simulink model "motor_io_velocity"  (R2014b)
settings: Solver=ode1  StartTime=0.0  StopTime=inf  FixedStep=Ts  RelTol=1e-3
PostLoadFcn:
  | , if any(exist('dsrtsu_mdlpostloadfcn', 'file') == [2, 3, 6]), try dsrtsu_mdlpostloadfcn('Execute', bdroot); catch fprintf('Error in PostLoadFcn (dsrtsu_mdlpostloadfcn) for model "%s":\n %s\n', bdroot, lasterr); end, end,
values from neighbouring files (symbols this model uses):
  F_c = 1.5e-3    (= 0.0015)    [continuous_design.m]    (also in workshop1.m)
  Gfb_d = c2d(S/R, Ts, 'tustin')    [continuous_design.m]    (also in workshop1.m = minreal(c2d(S/R, Ts, 'tustin')))
  Gff_d = c2d(T/R, Ts, 'tustin')    [continuous_design.m]    (also in workshop1.m = minreal(c2d(T/R, Ts, 'tustin')))
  J1 = 0.0006    [continuous_design.m]    (also in workshop1.m)
  motor = motor_pars    [continuous_design.m]    (also in workshop1.m)
  n = 5    [continuous_design.m]    (also in workshop1.m)
  R_vector = [1 0]    [workshop1.m]
  S_vector = [s1 s2]    [workshop1.m]
  T_vector = t0*[1 omega2]    [workshop1.m]
  Ts = 2*pi/ws    (= 0.0199466200228)    [continuous_design.m]    (also in pbutest.m = 0.0108705628152; workshop1.m = Ts_p)
libraries: rtilib1104 x5, simulink x1
settings Model: DSRTSU_INTERNAL_RTI_VER=450  DSRTSU_INTERNAL_RTI_TYPE=rti1104  DSRTSU_INTERNAL_RTIFPGA=40  ExtModeArmWhenConnect=off  BufferReuse=off  Creator=user  LastModifiedBy=es2lab2
settings DataIOCC: SignalLoggingSaveFormat=ModelDataLogs  SaveOutput=off  SignalLoggingName=sigsOut
settings OptimizationCC: BlockReduction=off  ConditionallyExecuteInputs=off  OptimizeBlockIOStorage=off  BufferReuse=off  GlobalBufferReuse=off  ExpressionFolding=off  ExpressionDepthLimit=2147483647  LocalBlockOutputs=off  InitFltsAndDblsToZero=on
settings DebuggingCC: SaveWithParameterizedLinksMsg=none  UnderspecifiedInitializationDetection=Classic  MergeDetectMultiDrivingBlocksExec=none  SignalResolutionControl=TryResolveAllWithWarning  SolverPrmCheckMsg=none  MultiTaskDSMMsg=warning  MultiTaskCondExecSysMsg=none  FcnCallInpInsideContextMsg=UseLocalSettings  UnconnectedInputMsg=none  UnconnectedOutputMsg=none  StateNameClashWarn=warning
settings HardwareCC: ProdIntDivRoundTo=Zero  ProdEndianess=BigEndian  ProdHWDeviceType=Generic->Custom  TargetIntDivRoundTo=Zero  TargetEndianess=BigEndian  TargetHWDeviceType=Generic->Custom
settings RTWCC: SystemTargetFile=rti1104.tlc  MakeCommand=make_rti  TemplateMakefile=rti1104.tmf  Description=dSPACE DS1104 Hardware Platform  RetainRTWFile=on  ProcessScript=rti1104_make_rtw_hook  IncludeERTFirstTime=on
settings STFCustomTargetCC: TargetFcnLib=ansi_tfl_tmw.mat  ParMdlRefBuildCompliant=on  GeneratePreprocessorConditionals=Disable all  SystemTargetFile=rti1104.tlc
settings GRTTargetCC: TargetFcnLib=ansi_tfl_tmw.mat  CompOptLevelCompliant=off  ConcurrentExecutionCompliant=off  CombineOutputUpdateFcns=off  MatFileLogging=off  CPPClassGenCompliant=off  GRTInterface=on  ExtModeMexFile=noextcomm

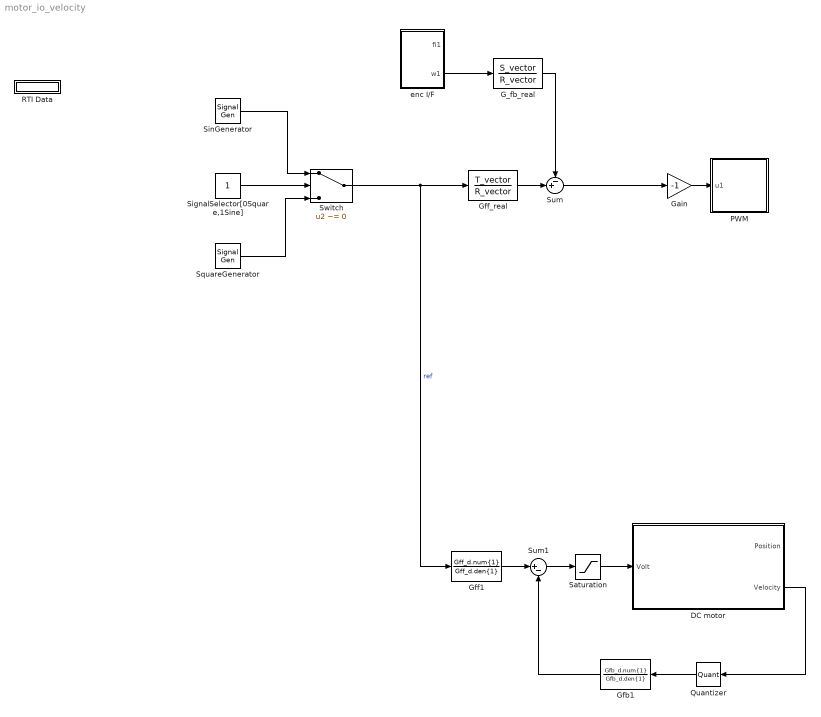
== system motor_io_velocity ==
  DC motor : Subsystem
  G_fb_real : DiscreteTransferFcn  Numerator=S_vector  Denominator=R_vector  SampleTime=Ts
  Gain : Gain  Gain=-1
  Gfb1 : DiscreteTransferFcn  Numerator=Gfb_d.num{1}  Denominator=Gfb_d.den{1}  SampleTime=Ts
  Gff1 : DiscreteTransferFcn  Numerator=Gff_d.num{1}  Denominator=Gff_d.den{1}  SampleTime=Ts
  Gff_real : DiscreteTransferFcn  Numerator=T_vector  Denominator=R_vector  SampleTime=Ts
  PWM : Subsystem
  Quantizer : Quantizer  QuantizationInterval=quant
  RTI Data : Subsystem  Tag=struct('RTIDataServer',struct('RTIDataServerVs','2','RTIModelDescription','struct(''main'',''motor_io_velocity'',''sub'','''',''isMp'',0)'))  LoadFcn="if exist('rtidc'), try,  rtidc('DataHostBlockClbLoad', gcbh); catch, disp(['Warning: ''LoadFcn'' for RTI Data block failed: ' lasterr]); end, end,"  mask(RTI_DATA_HOST){}
      mask help:
      | RTI Data Block.
      | This block is used by RTI to store internal model-dependent data.
      | Please keep this block on the root level of the model. Deleting this block will result in data loss.
      |
      | NEVER DELETE OR COPY THIS BLOCK!
      settings: CopyFcn="if exist('rtidc'), try,  rtidc('DataHostBlockClbCopy', gcbh); catch, disp(['Warning: ''CopyFcn'' for RTI Data block failed: ' lasterr]); end, end,"  DeleteFcn="if exist('rtidc'), try,  rtidc('DataHostBlockClbDelete', gcbh); catch, disp(['Warning: ''DeleteFcn'' for RTI Data block failed: ' lasterr]); end, end,"  ModelCloseFcn="if exist('rtidc'), try,  rtidc('DataHostBlockClbModelClose', gcbh); catch, disp(['Warning: ''ModelCloseFcn'' for RTI Data block failed: ' lasterr]); end, end,"  PreSaveFcn="if exist('rtidc'), try,  rtidc('DataHostBlockClbPreSave', gcbh); catch, disp(['Warning: ''PreSaveFcn'' for RTI Data block failed: ' lasterr]); end, end,"  PostSaveFcn="if exist('rtidc'), try,  rtidc('DataHostBlockClbPostSave', gcbh); catch, disp(['Warning: ''PostSaveFcn'' for RTI Data block failed: ' lasterr]); end, end,"  NameChangeFcn="if exist('rtidc'), try,  rtidc('DataHostBlockClbNameChange', gcbh); catch, disp(['Warning: ''NameChangeFcn'' for RTI Data block failed: ' lasterr]); end, end,"
      mask Help:
      | RTI Data Block.
      | This block is used by RTI to store internal model-dependent data.
      | Please keep this block on the root level of the model. Deleting this block will result in data loss.
      | 
      | NEVER DELETE OR COPY THIS BLOCK!
      mask Display:
      | text(0.5, 0.5, 'RTI Data', 'HorizontalAlignment', 'center');
      | plot([1 0]);
  Saturation : Saturate  UpperLimit=24  LowerLimit=-24
  SignalSelector[0Square,1Sine] : Constant
  SinGenerator : SignalGenerator  Amplitude=0  Units=rad/sec
  SquareGenerator : SignalGenerator  WaveForm=square  Amplitude=0  Units=rad/sec
  Sum : Sum  Inputs=-+|
  Sum1 : Sum  Inputs=|+-
  Switch : Switch  Criteria=u2 ~= 0
  enc I/F : Subsystem
  wires:
  SinGenerator/1 -> Switch/1
  SquareGenerator/1 -> Switch/3
  SignalSelector[0Square,1Sine]/1 -> Switch/2
  Gain/1 -> PWM/1(u1)
  Switch/1 -> Gff1/1, Gff_real/1  "ref"
  ? -> ?
  Gff_real/1 -> Sum/2
  Gff1/1 -> Sum1/1
  Sum1/1 -> Saturation/1
  Sum/1 -> Gain/1
  Gfb1/1 -> Sum1/2
  DC motor/2(Velocity) -> Quantizer/1
  enc I/F/2(w1) -> G_fb_real/1
  G_fb_real/1 -> Sum/1
  Saturation/1 -> DC motor/1(Volt)
  Quantizer/1 -> Gfb1/1

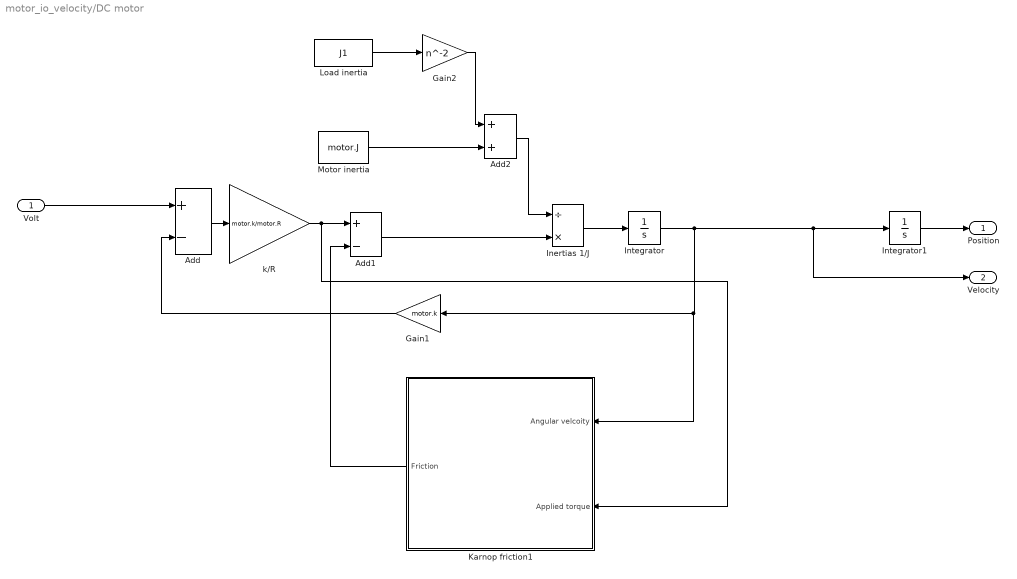
== system motor_io_velocity/DC motor ==
  Volt : Inport
  Add : Sum  Inputs=+-
  Add1 : Sum  Inputs=+-
  Add2 : Sum
  Gain1 : Gain  Gain=motor.k
  Gain2 : Gain  Gain=n^-2
  Inertias 1/J : Product  Inputs=/*
  Integrator : Integrator
  Integrator1 : Integrator
  Karnop friction1 : Subsystem
  Load inertia : Constant  Value=J1
  Motor inertia : Constant  Value=motor.J
  "k/R " : Gain  Gain=motor.k/motor.R
  Position : Outport
  Velocity : Outport  Port=2
  wires:
  Gain1/1 -> Add/2
  Add/1 -> "k/R "/1
  "k/R "/1 -> Karnop friction1/2(Applied torque), Add1/1
  Inertias 1/J/1 -> Integrator/1
  Integrator1/1 -> Position/1
  Add1/1 -> Inertias 1/J/2
  Volt/1 -> Add/1
  Integrator/1 -> Karnop friction1/1(Angular velcoity), Gain1/1, Velocity/1, Integrator1/1
  Motor inertia/1 -> Add2/2
  Load inertia/1 -> Gain2/1
  Gain2/1 -> Add2/1
  Add2/1 -> Inertias 1/J/1
  Karnop friction1/1(Friction) -> Add1/2

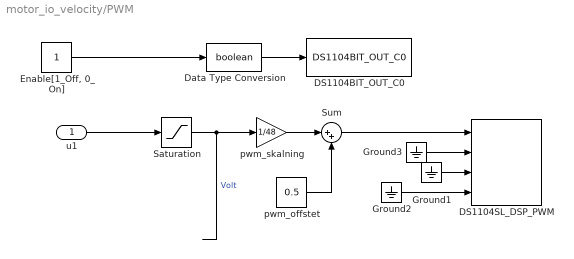
== system motor_io_velocity/PWM ==
  u1 : Inport
  DS1104BIT_OUT_C0 : rtilib1104/DS1104 MASTER PPC/DS1104BIT_OUT_C0  ChannelNo=0  InitValue=1  TermMode=0  TermValue=0  Reserved1=[]  Reserved2=[]  Reserved3=[]  Reserved=[]  DialogFcn=gui1104bit_out  UnitName={'DS1104BIT_OUT_C'}  UnitValues={ 0 }  DSProperties=struct('RTI',struct('Version',uint32(1),'BlockType',struct('isSLSource',uint8(0),'isSLSink',uint8(1),'isHWSource',uint8(0),'isHWSink',uint8(1),'isSetup',uint8(0),'isInline',uint8(1),'isNonInline',uint8(0),'isInterrupt',uint8(0),'isChannelwise',uint8(1)),'IOBoardType','DS1104MASTER','UnitType','BIT','Identifier','BITOUTCH','DialogType','ML','BlockSet','NONE','SlaveProcessor','NONE'))
  DS1104SL_DSP_PWM : rtilib1104/DS1104 SLAVE DSP/DS1104SL_DSP_PWM  Parameters=[]  TDef=[]  BoardType=[]  PwmMode=1  Frequency=20000  InitValue=[0.5 0.5 0.5 0.5]  TermMode=[0 0 0 0]  TermValue=[0.5 0.5 0.5 0.5]  Polarity=[1 1 1 1]  DialogFcn=gui1104sl_dsp_pwm  Reserved1=[]  Reserved2=[]  Reserved3=[]  Reserved4=[]  Revision=[]  UnitName={'DS1104SL_DSP_PWM'}  UnitValues={[]}  DSProperties=struct('RTI',struct('Version',uint32(2),'BlockType',struct('isSLSource',uint8(0),'isSLSink',uint8(1),'isHWSource',uint8(0),'isHWSink',uint8(1),'isSetup',uint8(0),'isInline',uint8(1),'isNonInline',uint8(0),'isInterrupt',uint8(0),'isChannelwise',uint8(0)),'IOBoardType','DS1104SLAVE','UnitType','PWM','Identifier','PWM','DialogType','ML','BlockSet','NONE','SlaveProcessor','F240'))  RTIBlockInterface=struct('InputPortsActive',[1 1 1 1],'InputPortsWidth',int32([1 1 1 1]),'InputPortsName',{{['PWM Channel 1'],['PWM Channel 2'],['PWM Channel 3'],['PWM Channel 4']}},'IWork',{{{'',uint32(4)}}},'DialogFcn','rti1104slavepwmgui','InitLevel',1,'BlockDisplay',{{'','auto'}},'IconTransparency','on','MultiSFcn',4,'BlockName',struct('Token',{{'DS1104SL_DSP_PWM'}}))  RTIBlockParameters=struct('PWMSymmetryMode',{{1,'OFF',[]}},'PWMFrequency',{{'50000','OFF',[]}},'PWMPolarityMode',{{[1 1 1 1 1],'OFF',[]}},'ChannelNo',{{[1 2 3 4],'OFF',[]}},'SuspendModeInit',{{[0 0 0 0 1],'OFF',[]}},'TTLModeInit',{{[2 2 2 2 2],'OFF',[]}},'DutyCycleInitValueCh1',{{'0.5','OFF',[]}},'DutyCycleInitValueCh2',{{'0.5','OFF',[]}},'DutyCycleInitValueCh3',{{'0.5','OFF',[]}},'DutyCycleInitValueCh4',{{'0.5','OFF',[]}},'DutyCycleInitValueCh5',{{'0.5','OFF',[]}},'EnablePWMStop',{{[0 0 0 0 0],'OFF',[]}},'SuspendModeTerm',{{[0 0 0 0 1],'OFF',[]}},'TTLModeTerm',{{[2 2 2 2 2],'OFF',[]}},'DutyCycleTermValueCh1',{{'0.5','OFF',[]}},'DutyCycleTermValueCh2',{{'0.5','OFF',[]}},'DutyCycleTermValueCh3',{{'0.5','OFF',[]}},'DutyCycleTermValueCh4',{{'0.5','OFF',[]}},'DutyCycleTermValueCh5',{{'0.5','OFF',[]}},'TLCFileName',{{'rti1104pwm','OFF',[]}})  RTISFcnParameters=struct('PWMSymmetryMode','double','PWMFrequency','double','PWMPolarityMode','double','ChannelNo','double','SuspendModeInit','double','TTLModeInit','double','DutyCycleInitValueCh1','double','DutyCycleInitValueCh2','double','DutyCycleInitValueCh3','double','DutyCycleInitValueCh4','double','EnablePWMStop','double','SuspendModeTerm','double','TTLModeTerm','double','DutyCycleTermValueCh1','double','DutyCycleTermValueCh2','double','DutyCycleTermValueCh3','double','DutyCycleTermValueCh4','double','TLCFileName','char')  RTIBlockParaDefault=struct('PWMSymmetryMode',1,'PWMFrequency',100,'PWMPolarityMode',[1 1 1 1 1],'ChannelNo',[1 2 3 4],'SuspendModeInit',[1 1 1 1 1],'TTLModeInit',[2 2 2 2 2],'DutyCycleInitValueCh1',0.5,'DutyCycleInitValueCh2',0.5,'DutyCycleInitValueCh3',0.5,'DutyCycleInitValueCh4',0.5,'DutyCycleInitValueCh5',0.5,'EnablePWMStop',[1 1 1 1 0],'SuspendModeTerm',[1 1 1 1 1],'TTLModeTerm',[2 2 2 2 2],'DutyCycleTermValueCh1',0.5,'DutyCycleTermValueCh2',0.5,'DutyCycleTermValueCh3',0.5,'DutyCycleTermValueCh4',0.5,'DutyCycleTermValueCh5',0.5,'TLCFileName','rti1104pwm')
  Data Type Conversion : DataTypeConversion  OutDataTypeStr=boolean  SaturateOnIntegerOverflow=on  RndMeth=Zero
  "Enable[1_Off, 0_On]" : Constant
  Ground1 : Ground
  Ground2 : Ground
  Ground3 : Ground
  Saturation : Saturate  UpperLimit=24  LowerLimit=-24
  Sum : Sum  Inputs=|++  SaturateOnIntegerOverflow=on
  pwm_offstet : Constant  Value=0.5
  pwm_skalning : Gain  Gain=1/48  SaturateOnIntegerOverflow=on  OutDataTypeStr=Inherit: Same as input  ParamDataTypeStr=Inherit: Same as input
  wires:
  "Enable[1_Off, 0_On]"/1 -> Data Type Conversion/1
  Data Type Conversion/1 -> DS1104BIT_OUT_C0/1
  pwm_skalning/1 -> Sum/1
  Sum/1 -> DS1104SL_DSP_PWM/1
  pwm_offstet/1 -> Sum/2
  u1/1 -> Saturation/1
  Ground1/1 -> DS1104SL_DSP_PWM/3
  Ground2/1 -> DS1104SL_DSP_PWM/4
  Ground3/1 -> DS1104SL_DSP_PWM/2
  Saturation/1 -> pwm_skalning/1  "Volt"

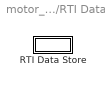
== system motor_io_velocity/RTI Data ==
  RTI Data Store : Subsystem  Tag="struct('public',struct('sub',struct('name',{{'motor_io_velocity'}},'data',{{struct('TH',struct('thTaskInfo',struct('taskType',{'TIMER','HWINT','TMRINT','SWINT','GLINT'},'tasksNumOf',{1,0,0,0,0},'srcIds',{{'TIMERA'},{},{},{},{}},'taskNames',{{['Timer Task 1']},{},{},{},{}})),'th_tc',struct('dataType','TASK','taskGroupId','','taskGroupList',{{}},'taskSchedulingPolicy','FCFS','taskType','TIMER','blkh',-1,'srcId','TIMERA','srcSgnName',['Timer A interrupt'],'srcCpuName','','taskName',['Timer Task 1  [0.0219701] s'],'taskNameDisplayExt','','smplTime',0.021970064966318436,'smplTimeOffs',0,'hasFixedPriority',0,'priority',1,'hasFixedOvc',0,'ovcType',1,'ovcMax',1),'tc_th',struct('dataType','TASK','taskGroupId','','taskGroupList',{{}},'taskSchedulingPolicy','FCFS','taskType','TIMER','blkh',-1,'srcId','TIMERA','srcSgnName',['Timer A interrupt'],'srcCpuName','','taskName',['Timer Task 1  [0.0219701] s'],'taskNameDisplayExt','','smplTime',0.021970064966318436,'smplTimeOffs',0,'hasFixedPriority',0,'priority',1,'hasFixedOvc',0,'ovcType',1,'ovcMax',1))}})),'private',struct('version',struct('dsVer',uint32(2)),'access',struct('modified',['30-Mar-2016 14:28:40'],'type','Model','isPerm',1)))"  mask(RTI_DATA_STORE){}
      mask help:
      | RTI Data Store Block. This block is used by RTI to store internal model dependent data. Deleting this block will result in data loss.
      |
      | NEVER DELETE, COPY, OR MODIFY THIS BLOCK!
      mask Help:
      | RTI Data Store Block. This block is used by RTI to store internal model dependent data. Deleting this block will result in data loss.
      | 
      | NEVER DELETE, COPY, OR MODIFY THIS BLOCK!
      mask Display: text(0.5, 0.5, ' ', 'HorizontalAlignment', 'center');

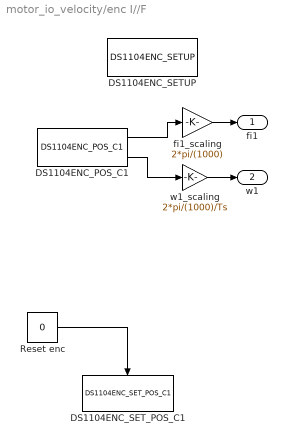
== system motor_io_velocity/enc I//F ==
  DS1104ENC_POS_C1 : rtilib1104/DS1104 MASTER PPC/DS1104ENC_POS_C1  ChannelNo=1  PosValue=0  Reserved1=[]  Reserved2=[]  Reserved3=[]  Reserved4=[]  DialogFcn=gui1104enc_pos  UnitName={'DS1104ENC_POS_C'}  UnitValues={ 1 }  DSProperties=struct('RTI',struct('Version',uint32(1),'BlockType',struct('isSLSource',uint8(1),'isSLSink',uint8(0),'isHWSource',uint8(1),'isHWSink',uint8(0),'isSetup',uint8(0),'isInline',uint8(1),'isNonInline',uint8(0),'isInterrupt',uint8(0),'isChannelwise',uint8(1)),'IOBoardType','DS1104MASTER','UnitType','ENC','Identifier','ENCPOSCH','DialogType','ML','BlockSet','NONE','SlaveProcessor','NONE'))
  DS1104ENC_SETUP : rtilib1104/DS1104 MASTER PPC/DS1104ENC_SETUP  Reserved1=[]  Reserved2=[]  Reserved3=[]  Reserved4=[]  DialogFcn=gui1104enc_setup  UnitName={'DS1104ENC_SETUP'}  UnitValues={ [] }  DSProperties=struct('RTI',struct('Version',uint32(1),'BlockType',struct('isSLSource',uint8(0),'isSLSink',uint8(0),'isHWSource',uint8(0),'isHWSink',uint8(0),'isSetup',uint8(0),'isInline',uint8(1),'isNonInline',uint8(0),'isInterrupt',uint8(0),'isChannelwise',uint8(0)),'IOBoardType','DS1104MASTER','UnitType','ENC','Identifier','ENCSETUP','DialogType','ML','BlockSet','NONE','SlaveProcessor','NONE'))
      settings: SignalType=[1 0]
  DS1104ENC_SET_POS_C1 : rtilib1104/DS1104 MASTER PPC/DS1104ENC_SET_POS_C1  ChannelNo=1  PosValue=0  Reserved1=[]  Reserved2=[]  Reserved3=[]  Reserved4=[]  DialogFcn=gui1104enc_set_pos  UnitName={'DS1104ENC_SET_POS_C'}  UnitValues={ 1 }  DSProperties=struct('RTI',struct('Version',uint32(1),'BlockType',struct('isSLSource',uint8(0),'isSLSink',uint8(1),'isHWSource',uint8(0),'isHWSink',uint8(1),'isSetup',uint8(0),'isInline',uint8(1),'isNonInline',uint8(0),'isInterrupt',uint8(0),'isChannelwise',uint8(1)),'IOBoardType','DS1104MASTER','UnitType','ENC','Identifier','ENCRESET','DialogType','ML','BlockSet','NONE','SlaveProcessor','NONE'))
  Reset enc : Constant  Value=0
  fi1_scaling : Gain  Gain=2*pi/(1000)  SaturateOnIntegerOverflow=on  OutDataTypeStr=Inherit: Same as input  ParamDataTypeStr=Inherit: Same as input
  w1_scaling : Gain  Gain=2*pi/(1000)/Ts  SaturateOnIntegerOverflow=on  OutDataTypeStr=Inherit: Same as input  ParamDataTypeStr=Inherit: Same as input
  fi1 : Outport
  w1 : Outport  Port=2
  wires:
  Reset enc/1 -> DS1104ENC_SET_POS_C1/Trigger
  DS1104ENC_POS_C1/1 -> fi1_scaling/1
  DS1104ENC_POS_C1/2 -> w1_scaling/1
  fi1_scaling/1 -> fi1/1
  w1_scaling/1 -> w1/1

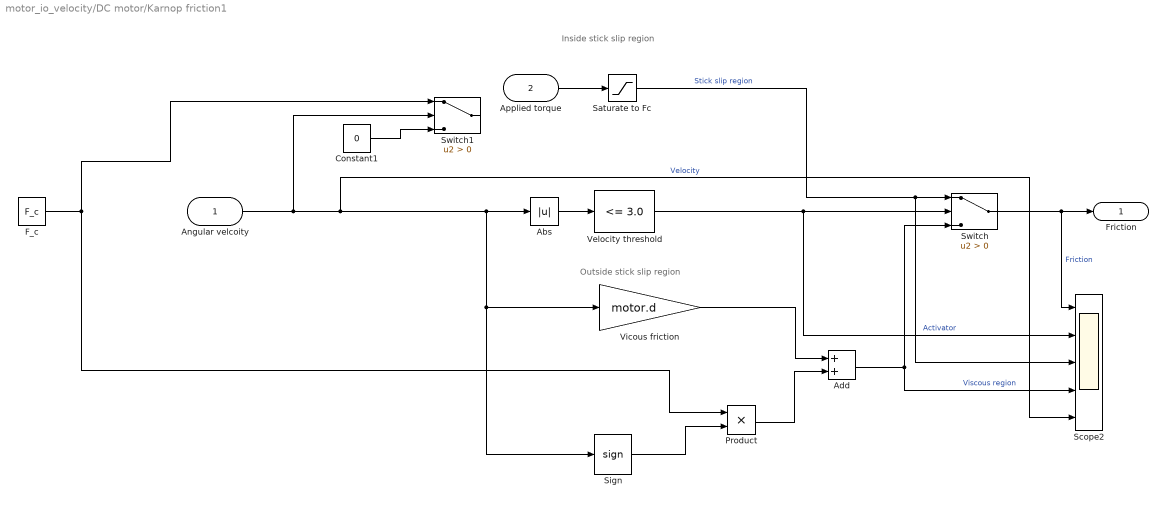
== system motor_io_velocity/DC motor/Karnop friction1 ==
  note: Inside stick slip region
  note: Outside stick slip region
  Angular velcoity : Inport
  Applied torque : Inport  Port=2
  Abs : Abs  ZeroCross=off
  Add : Sum
  Constant1 : Constant  Value=0
  F_c : Constant  Value=F_c
  Product : Product
  Saturate to Fc : Saturate  UpperLimit=F_c  LowerLimit=-F_c  ZeroCross=off
  Scope2 : Scope  NumInputPorts=5
      settings: ShowLegends=on  YMin=-0.00177~-0.125~0.0009~-0.00177~-138.1533~-0.12501~-0.12501~-0.12501  YMax=0.00177~1.125~0.0011~0.00177~138.10681~0.12501~0.12501~0.12501  SaveName=ScopeData3
  Sign : Signum  ZeroCross=off
  Switch : Switch  Criteria=u2 > Threshold  ZeroCross=off
  Switch1 : Switch  Criteria=u2 > Threshold  ZeroCross=off
  "Velocity threshold " : simulink/Logic and Bit Operations/Compare To Constant  relop=<=  const=3.0  OutDataTypeStr=boolean
  Vicous friction : Gain  Gain=motor.d
  Friction : Outport
  wires:
  Constant1/1 -> Switch1/3
  Saturate to Fc/1 -> Scope2/3, Switch/1  "Stick slip region"
  Switch/1 -> Scope2/1, Friction/1  "Friction"
  Angular velcoity/1 -> Scope2/5, Abs/1, Vicous friction/1, Sign/1, Switch1/2  "Velocity"
  "Velocity threshold "/1 -> Scope2/2, Switch/2  "Activator"
  Abs/1 -> "Velocity threshold "/1
  Product/1 -> Add/2
  Vicous friction/1 -> Add/1
  F_c/1 -> Switch1/1, Product/1
  Sign/1 -> Product/2
  Add/1 -> Switch/3, Scope2/4  "Viscous region"
  Applied torque/1 -> Saturate to Fc/1

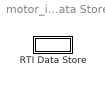
== system motor_io_velocity/RTI Data/RTI Data Store ==
  RTI Data Store : Subsystem  mask(RTI_DATA_STORE){}
      mask help:
      | RTI Data Store Block. This block is used by RTI to store internal model dependent data. Deleting this block will result in data loss.
      |
      | NEVER DELETE, COPY, OR MODIFY THIS BLOCK!
      mask Help:
      | RTI Data Store Block. This block is used by RTI to store internal model dependent data. Deleting this block will result in data loss.
      | 
      | NEVER DELETE, COPY, OR MODIFY THIS BLOCK!
      mask Display: text(0.5, 0.5, ' ', 'HorizontalAlignment', 'center');

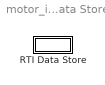
== system motor_io_velocity/RTI Data/RTI Data Store/RTI Data Store ==
  RTI Data Store : Subsystem  mask(RTI_DATA_STORE){}
      mask help:
      | RTI Data Store Block. This block is used by RTI to store internal model dependent data. Deleting this block will result in data loss.
      |
      | NEVER DELETE, COPY, OR MODIFY THIS BLOCK!
      mask Help:
      | RTI Data Store Block. This block is used by RTI to store internal model dependent data. Deleting this block will result in data loss.
      | 
      | NEVER DELETE, COPY, OR MODIFY THIS BLOCK!
      mask Display: text(0.5, 0.5, ' ', 'HorizontalAlignment', 'center');

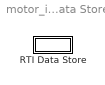
== system motor_io_velocity/RTI Data/RTI Data Store/RTI Data Store/RTI Data Store ==
  RTI Data Store : Subsystem  mask(RTI_DATA_STORE){}
      mask help:
      | RTI Data Store Block. This block is used by RTI to store internal model dependent data. Deleting this block will result in data loss.
      |
      | NEVER DELETE, COPY, OR MODIFY THIS BLOCK!
      mask Help:
      | RTI Data Store Block. This block is used by RTI to store internal model dependent data. Deleting this block will result in data loss.
      | 
      | NEVER DELETE, COPY, OR MODIFY THIS BLOCK!
      mask Display: text(0.5, 0.5, ' ', 'HorizontalAlignment', 'center');

== system motor_io_velocity/RTI Data/RTI Data Store/RTI Data Store/RTI Data Store/RTI Data Store ==
